simulink model "eg3"  (R2021a)
settings: Solver=ode1  StartTime=0  StopTime=10.0  FixedStep=0.001  RelTol=1e-6
settings Model: Creator=lilic  LastModifiedBy=Jieming

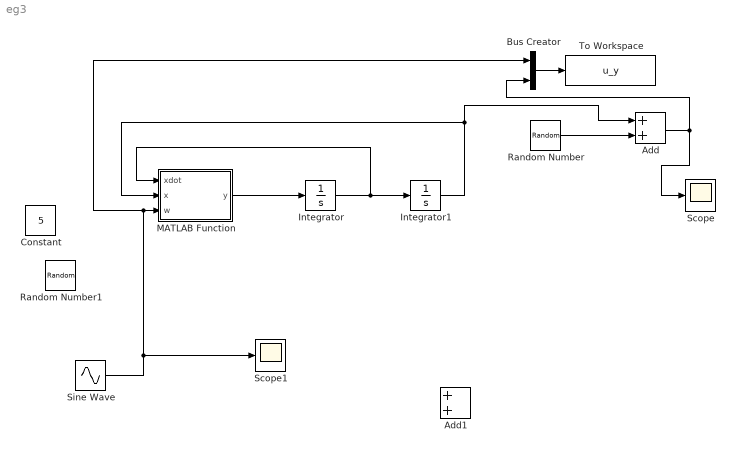
== system eg3 ==
  Add : Sum
  Add1 : Sum
  Bus Creator : BusCreator  Inputs=2
  Constant : Constant  Value=5
  Integrator : Integrator
  Integrator1 : Integrator  InitialCondition=1
  MATLAB Function : MATLAB Function  TreatAsAtomicUnit=on
  Random Number : RandomNumber  Variance=0
  Random Number1 : RandomNumber  Mean=5  Variance=0.000001
  Scope : Scope
  Scope1 : Scope
  Sine Wave : Sin  Amplitude=5  SampleTime=0
  To Workspace : ToWorkspace  VariableName=u_y  SaveFormat=Timeseries  SampleTime=-1
  wires:
  Integrator/1 -> MATLAB Function/1(xdot), Integrator1/1
  MATLAB Function/1(y) -> Integrator/1
  Integrator1/1 -> Add/1, MATLAB Function/2(x)
  Sine Wave/1 -> Bus Creator/1, MATLAB Function/3(w), Scope1/1
  Bus Creator/1 -> To Workspace/1
  Random Number/1 -> Add/2
  Add/1 -> Scope/1, Bus Creator/2

== matlab function eg3/MATLAB Function ==
  data: xdot input; y output; x input; w input
function y = fcn(xdot,x,w)
gamma=0.01;
epsilon=1;
delta=0;
y = -(gamma*xdot+w^2*x+epsilon*x^2*xdot+delta*xdot^3);
